simulink model "vehicle_hostmodel_2022b_v11"  (R2024b)
settings: Solver=ode4  StartTime=0.0  StopTime=inf  FixedStep=0.01  MaxStep=0.05  RelTol=1e-3
PreLoadFcn:
  | load("FInalGraph.mat")
model workspace (MAT data in the model file):
  G_final : digraph (value not decoded)
values from neighbouring files (symbols this model uses):
  ActorID = 0    [HelperSpeedActionAdapter.m]
  D = cross(B-A,C-A)    [HelperCalculateEgoRefPathInfo.m]
  L = zeros(N,1)    [HelperCalculateEgoRefPathInfo.m]
  psi_o = -1.185    [sensor.m]
  R = NaN(N,1)    [HelperCalculateEgoRefPathInfo.m]
  SceneInfo = [-32.1351766513 25.1612903226 -74.2242703533 -71.4592933948 -32.2887864823 26.2365591398 26.8509984639 27.0046082949 -32.7496159754 -72.380952381 -49.846390169 -49.3855606759 ... (30 elements, 10x3)]    [SceneLabels.mat]
  Ts = 0.05    [sensor.m]
undefined symbols (not defined in the file or in its folder): Acceleration, AngularVelocity, barrier_1, barrier_2, barrier_3, curvature, DefaultGear, DEND_B, DEND_S, DEND_T, direction, DiscIntNeverNeededParam, driving, finalint, goal1_coordinates, goal2_coordinates, goal3_coordinates, gradbp, latlongcoordinates, LF, LR, matlabshared, MAX_BRAKE, MAX_STEER, MAX_TORQUE, MCAR, MIN_BRAKE, MIN_STEER, MIN_TORQUE, NUMD_B, NUMD_S, NUMD_T, Pitch, Position, Roll, RRdamp, session, sigbuilder_block, STEER_RATIO, stopSign_ID, Tdead, thetaRefs, TL_ID, TrackWidth, ts, Vdead, Velocity, WB, xRef2s, Yaw, yRef2s
libraries: simulink x10, drivingscenarioandsensors x8, simulink_extras x4, drivingvehiclecontroller x2, trackingutilitieslib x2, robotalgslib x1, mpcadaslib x1, slpidlib x1, drivinglib x1, autolibshared x1, vehdynlibviscommon x1, vehdynlibsteering x1
(part 3 of 4)

== system vehicle_hostmodel_2022b_v11/Controllers/Subsystem2/Subsystem/Function-Call Subsystem ==
  CurrVelocity : Inport
  Relative Distance : Inport  Port=2
  function : TriggerPort  VariantControl=(inherit)  ShowOutputPort=on
  MATLAB Function1 : MATLAB Function  TreatAsAtomicUnit=on
  Saturation : Saturate  UpperLimit=0.3*9.8  LowerLimit=0
  BrakingAcc : Outport
  wires:
  CurrVelocity/1 -> MATLAB Function1/1(Vel)
  Relative Distance/1 -> MATLAB Function1/2(RelDist)
  MATLAB Function1/1(BrakingAcc) -> Saturation/1
  Saturation/1 -> BrakingAcc/1

== system vehicle_hostmodel_2022b_v11/Controllers/Subsystem2/Subsystem/Subsystem2 ==
  decc_cmd : Inport
  Constant1 : Constant  Value=MCAR
  Gain : Gain  Gain=1.1*MCAR
  Gain1 : Gain  Gain=1.2*0.3*2/2
  Gain2 : Gain  Gain=0.7*9.81
  Gain4 : Gain  Gain=-R/(7.05*0.8)
  Integrator : Integrator  ExternalReset=falling
  Square : Math  Operator=square
  Sum : Sum  Inputs=+++
  T_brake_cmd : Outport
  wires:
  Square/1 -> Gain1/1
  Integrator/1 -> Square/1  "v"
  Gain4/1 -> T_brake_cmd/1  "T_eng"
  Gain1/1 -> Sum/1  "F_aero"
  Gain2/1 -> Sum/2
  decc_cmd/1 -> Integrator/2, Integrator/1, Gain/1
  Sum/1 -> Gain4/1
  Gain/1 -> Sum/3
  Constant1/1 -> Gain2/1

== system vehicle_hostmodel_2022b_v11/Controllers/Subsystem2/Subsystem1/Subsystem2 ==
  acc_cmd : Inport
  decc_cmd : Inport  Port=2
  Subsystem : Subsystem
  Subsystem1 : Subsystem
  T_eng_cmd : Outport
  brake_cmd : Outport  Port=2
  wires:
  acc_cmd/1 -> Subsystem/1(acc_cmd)
  Subsystem/1(T_eng_cmd) -> T_eng_cmd/1
  decc_cmd/1 -> Subsystem1/1(decc_cmd)
  Subsystem1/1(T_brake_cmd) -> brake_cmd/1

== system vehicle_hostmodel_2022b_v11/Environment & Data/Sensors & Perception/Tracking/Subsystem1 ==
  In2 : Inport
  EgoV : Inport  Port=2
  Camera : drivingscenarioandsensors/Vision Detection Generator  SensorIndex=1  DetectorOutput=Objects only  UpdateInterval=0.1  LaneUpdateInterval=0.1  SensorLocation=[1.9 0]  Height=1.1  Yaw=0  Pitch=1  Roll=0  BusNameSource=Auto  BusName=BusObjectDetections  BusName2Source=Auto  BusName2=BusLaneDetections  MaxNumDetectionsSource=Property  MaxNumDetections=10  MaxNumLanesSource=Property  MaxNumLanes=30  DetectionCoordinates=Ego Cartesian  SimulateUsing=Interpreted execution  MaxRange=150  BoundingBoxAccuracy=5  ProcessNoiseIntensity=5  MaxSpeed=100  MaxAllowedOcclusion=0.5  MinObjectImageSize=[5 5]  DetectionProbability=0.9  FalsePositivesPerImage=0.1  MinLaneImageSize=[20 3]  LaneBoundaryAccuracy=3  HasNoise=on  InitialSeedSource=Repeatable  InitialSeed=0  UsedSeed=0  ActorProfilesSource=From Scenario Reader block  ActorProfilesParameters=driving.internal.ActorProfilesParameters  ActorProfilesExpression=[struct('ActorID',1,'ClassID',1,'Length',4.7,'Width',1.8,'Height',1.4,'OriginOffset',[-1.35 0 0],'MeshVertices',[3.7 0.9 0.857439446366782;3.7 -0.9 0.857439446366782;3.7 -0.9 0.314878892733564;3.7 0.9 0.314878892733564;3.7 0.9 0.857439446366782;2.525 0.9 0.993079584775086;2.525 -0.9 0.993079584775086;3.7 -0.9 0.857439446366782;1.82 0.72 1.4;0.41 0.72 1.4;0.41 -0.72 1.4;1.82 -0.72 1.4;-0.295 0.9 0.993079584775086;-1 0.9 0.857439446366782;-1 -0.9 0.857439446366782;-0.295 -0.9 0.993079584775086;3.7 0.9 0.857439446366782;3.7 0.9 0.314878892733564;2.525 0.9 0.314878892733564;2.525 0.9 0.993079584775086;2.525 0.9 0.993079584775086;2.525 0.9 0.314878892733564;-0.295 0.9 0.314878892733564;-0.295 0.9 0.993079584775086;-0.295 0.9 0.993079584775086;-0.295 0.9 0.314878892733564;-1 0.9 0.355570934256055;-1 0.9 0.857439446366782;2.525 0.9 0.993079584775086;-0.295 0.9 0.993079584775086;0.41 0.72 1.4;1.82 0.72 1.4;3.7 -0.9 0.857439446366782;3.7 -0.9 0.314878892733564;2.525 -0.9 0.314878892733564;2.525 -0.9 0.993079584775086;2.525 -0.9 0.993079584775086;2.525 -0.9 0.314878892733564;-0.295 -0.9 0.314878892733564;-0.295 -0.9 0.993079584775086;-0.295 -0.9 0.993079584775086;-0.295 -0.9 0.314878892733564;-1 -0.9 0.355570934256055;-1 -0.9 0.857439446366782;2.525 -0.9 0.993079584775086;-0.295 -0.9 0.993079584775086;0.41 -0.72 1.4;1.82 -0.72 1.4;-0.295 0.9 0.993079584775086;-0.295 -0.9 0.993079584775086;0.41 -0.72 1.4;0.41 0.72 1.4;2.525 -0.9 0.993079584775086;1.82 -0.72 1.4;1.82 0.72 1.4;2.525 0.9 0.993079584775086;-1 0.9 0.857439446366782;-1 0.9 0.355570934256055;-1 -0.9 0.355570934256055;-1 -0.9 0.857439446366782;3.7 0.9 0.314878892733564;3.7 -0.9 0.314878892733564;-0.295 -0.9 0.314878892733564;-0.295 0.9 0.314878892733564;-0.295 0.9 0.314878892733564;-1 0.9 0.355570934256055;-1 -0.9 0.355570934256055;-0.295 -0.9 0.314878892733564;0 -0.63 0;0 -0.87 0;0.191030206995054 -0.63 0.0601365173421445;0.191030206995054 -0.87 0.0601365173421445;0.309093367795925 -0.63 0.217575963708927;0.309093367795925 -0.87 0.217575963708927;0.309093367795925 -0.63 0.412181821758201;0.309093367795925 -0.87 0.412181821758201;0.191030206995054 -0.63 0.569621268124983;0.191030206995054 -0.87 0.569621268124983;0 -0.63 0.629757785467128;0 -0.87 0.629757785467128;-0.191030206995054 -0.63 0.569621268124983;-0.191030206995054 -0.87 0.569621268124983;-0.309093367795925 -0.63 0.412181821758201;-0.309093367795925 -0.87 0.412181821758201;-0.309093367795925 -0.63 0.217575963708927;-0.309093367795925 -0.87 0.217575963708927;-0.191030206995054 -0.63 0.0601365173421445;-0.191030206995054 -0.87 0.0601365173421445;0 -0.63 0;0 -0.87 0;0 -0.63 0;0.191030206995054 -0.63 0.0601365173421445;0.309093367795925 -0.63 0.217575963708927;0.309093367795925 -0.63 0.412181821758201;0.191030206995054 -0.63 0.569621268124983;0 -0.63 0.629757785467128;-0.191030206995054 -0.63 0.569621268124983;-0.309093367795925 -0.63 0.412181821758201;-0.309093367795925 -0.63 0.217575963708927;-0.191030206995054 -0.63 0.0601365173421445;0 -0.87 0;0.191030206995054 -0.87 0.0601365173421445;0.309093367795925 -0.87 0.217575963708927;0.309093367795925 -0.87 0.412181821758201;0.191030206995054 -0.87 0.569621268124983;0 -0.87 0.629757785467128;-0.191030206995054 -0.87 0.569621268124983;-0.309093367795925 -0.87 0.412181821758201;-0.309093367795925 -0.87 0.217575963708927;-0.191030206995054 -0.87 0.0601365173421445;0 0.87 0;0 0.63 0;0.191030206995054 0.87 0.0601365173421445;0.191030206995054 0.63 0.0601365173421445;0.309093367795925 0.87 0.217575963708927;0.309093367795925 0.63 0.217575963708927;0.309093367795925 0.87 0.412181821758201;0.309093367795925 0.63 0.412181821758201;0.191030206995054 0.87 0.569621268124983;0.191030206995054 0.63 0.569621268124983;0 0.87 0.629757785467128;0 0.63 0.629757785467128;-0.191030206995054 0.87 0.569621268124983;-0.191030206995054 0.63 0.569621268124983;-0.309093367795925 0.87 0.412181821758201;-0.309093367795925 0.63 0.412181821758201;-0.309093367795925 0.87 0.217575963708927;-0.309093367795925 0.63 0.217575963708927;-0.191030206995054 0.87 0.0601365173421445;-0.191030206995054 0.63 0.0601365173421445;0 ...(+3718 chars)],'MeshFaces',[1 2 3;3 4 1;5 6 7;7 8 5;9 10 11;11 12 9;13 14 15;15 16 13;17 18 19;19 20 17;21 22 23;23 24 21;25 26 27;27 28 25;29 30 31;31 32 29;33 34 35;35 36 33;37 38 39;39 40 37;41 42 43;43 44 41;45 46 47;47 48 45;49 50 51;51 52 49;53 54 55;55 56 53;57 58 59;59 60 57;61 62 63;63 64 61;65 66 67;67 68 65;69 71 72;72 70 69;71 73 74;74 72 71;73 75 76;76 74 73;75 77 78;78 76 75;77 79 80;80 78 77;79 81 82;82 80 79;81 83 84;84 82 81;83 85 86;86 84 83;85 87 88;88 86 85;87 89 90;90 88 87;91 92 93;91 93 94;91 94 95;91 95 96;91 96 97;91 97 98;91 98 99;91 99 100;101 102 103;101 103 104;101 104 105;101 105 106;101 106 107;101 107 108;101 108 109;101 109 110;111 113 114;114 112 111;113 115 116;116 114 113;115 117 118;118 116 115;117 119 120;120 118 117;119 121 122;122 120 119;121 123 124;124 122 121;123 125 126;126 124 123;125 127 128;128 126 125;127 129 130;130 128 127;129 131 132;132 130 129;133 134 135;133 135 136;133 136 137;133 137 138;133 138 139;133 139 140;133 140 141;133 141 142;143 144 145;143 145 146;143 146 147;143 147 148;143 148 149;143 149 150;143 150 151;143 151 152;153 155 156;156 154 153;155 157 158;158 156 155;157 159 160;160 158 157;159 161 162;162 160 159;161 163 164;164 162 161;163 165 166;166 164 163;165 167 168;168 166 165;167 169 170;170 168 167;169 171 172;172 170 169;171 173 174;174 172 171;175 176 177;175 177 178;175 178 179;175 179 180;175 180 181;175 181 182;175 182 183;175 183 184;185 186 187;185 187 188;185 188 189;185 189 190;185 190 191;185 191 192;185 192 193;185 193 194;195 197 198;198 196 195;197 199 200;200 198 197;199 201 202;202 200 199;201 203 204;204 202 201;203 205 206;206 204 203;205 207 208;208 206 205;207 209 210;210 208 207;209 211 212;212 210 209;211 213 214;214 212 211;213 215 216;216 214 213;217 218 219;217 219 220;217 220 221;217 221 222;217 222 223;217 223 224;217 224 225;217 225 226;227 228 229;227 229 230;227 230 231;227 231 232;227 232 233;227 233 234;227 234 235;227 235 236],'RCSPattern',[10 10;10 10],'RCSAzimuthAngles',[-180 180],'RCSElevationAngles',[-90 90]); struct('ActorID',2,'ClassID',7,'Length',0.7,'Width',0.2,'Height',0.1,'OriginOffset',[0 0 0],'MeshVertices',[0.35 -0.1 0.1;0.35 0.1 0.1;-0.35 0.1 0.1;-0.35 -0.1 0.1;0.35 -0.1 0;0.35 0.1 0;-0.35 0.1 0;-0.35 -0.1 0],'MeshFaces',[6 2 1;1 5 6;8 4 3;3 7 8;6 7 3;3 2 6;5 1 4;4 8 5;4 1 2;2 3 4;7 6 5;5 8 7],'RCSPattern',[10 10;10 10],'RCSAzimuthAngles',[-180 180],'RCSElevationAngles',[-90 90])]  Intrinsics=driving.internal.cameraIntrinsics('FocalLength',[800 800],'PrincipalPoint',[320 240],'ImageSize',[480 640],'RadialDistortion',[0 0],'TangentialDistortion',[0 0],'Skew',0)
  Detection Concatenation : trackingutilitieslib/Detection Concatenation  NumInputs=3  BusNameSource=Auto  BusName=BusDetectionConcatenation  SimulateUsing=Interpreted execution
  Lidar Point Cloud Generator : drivingscenarioandsensors/Lidar Point Cloud Generator  SensorIndex=2  UpdateInterval=0.1  SensorLocation=[1.5 0]  Height=1.6  Yaw=0  Pitch=0  Roll=0  DetectionCoordinates=Ego Cartesian  HasEgoVehicle=on  EgoVehicleActorID=1  HasRoadsInputPort=on  ActorProfilesSource=From Scenario Reader block  ActorProfilesVariableName=actor_profiles  MaxRange=120  RangeAccuracy=0.002  AzimuthResolution=0.16  ElevationResolution=1.25  AzimuthLimits=[-60 60]  ElevationLimits=[ -20, 20 ]  HasNoise=on
  Lidar Point Cloud Generator1 : drivingscenarioandsensors/Lidar Point Cloud Generator  SensorIndex=3  UpdateInterval=0.1  SensorLocation=[1.5 0]  Height=1.6  Yaw=0  Pitch=0  Roll=0  DetectionCoordinates=Ego Cartesian  HasEgoVehicle=on  EgoVehicleActorID=1  HasRoadsInputPort=on  ActorProfilesSource=From Scenario Reader block  ActorProfilesVariableName=actor_profiles  MaxRange=120  RangeAccuracy=0.002  AzimuthResolution=0.16  ElevationResolution=1.25  AzimuthLimits=[60 180]  ElevationLimits=[ -20, 20 ]  HasNoise=on
  Lidar Point Cloud Generator2 : drivingscenarioandsensors/Lidar Point Cloud Generator  SensorIndex=4  UpdateInterval=0.1  SensorLocation=[1.5 0]  Height=1.6  Yaw=0  Pitch=0  Roll=0  DetectionCoordinates=Ego Cartesian  HasEgoVehicle=on  EgoVehicleActorID=1  HasRoadsInputPort=on  ActorProfilesSource=From Scenario Reader block  ActorProfilesVariableName=actor_profiles  MaxRange=120  RangeAccuracy=0.002  AzimuthResolution=0.16  ElevationResolution=1.25  AzimuthLimits=[-180 -60]  ElevationLimits=[ -20, 20 ]  HasNoise=on
  Camera Detections : Outport
  Radar detections : Outport  Port=2
  wires:
  EgoV/1 -> Lidar Point Cloud Generator1/2, Lidar Point Cloud Generator/2, Lidar Point Cloud Generator2/2
  Lidar Point Cloud Generator1/1 -> Detection Concatenation/2  "Lidar Detections"
  Lidar Point Cloud Generator2/1 -> Detection Concatenation/3  "Lidar Detections"
  Detection Concatenation/1 -> Radar detections/1
  Camera/1 -> Camera Detections/1  "Camera Detections"
  In2/1 -> Camera/1, Lidar Point Cloud Generator/1, Lidar Point Cloud Generator1/1, Lidar Point Cloud Generator2/1
  Lidar Point Cloud Generator/1 -> Detection Concatenation/1  "Lidar Detections"

== system vehicle_hostmodel_2022b_v11/Environment & Data/Visualisation & Data/Positions and States /Traffic Light Sensor ==
  note: Traffic Light Sensor
  TL_id : Inport
  Bus Creator : BusCreator  Inputs=2
  LightConfiguration : Constant  Value=TrafficLightSensorModeSelection
  Traffic Light Switching Logic : Stateflow chart  TreatAsAtomicUnit=on
  TL_State : Outport
  wires:
  LightConfiguration/1 -> Traffic Light Switching Logic/1(LightConfig)
  TL_id/1 -> Traffic Light Switching Logic/2(TL_id)
  Bus Creator/1 -> TL_State/1
  Traffic Light Switching Logic/2(trafficLight) -> Bus Creator/1
  Traffic Light Switching Logic/1(TL_ID) -> Bus Creator/2

== system vehicle_hostmodel_2022b_v11/Reference Data1/Subsystem1/Subsystem2/Subsystem ==
  note: Select method to calculate theta
  Integrator : Inport
  Curvature : Lookup_n-D  NumberOfTableDimensions=1  BreakpointsForDimension1=gradbp  Table=curvature  InternalRulePriority=Speed  RndMeth=Simplest
  Direction : Lookup_n-D  NumberOfTableDimensions=1  BreakpointsForDimension1=gradbp  Table=direction  InternalRulePriority=Speed  RndMeth=Simplest
  From Workspace1 : FromWorkspace  VariableName=yRef2  SampleTime=-1
  From Workspace2 : FromWorkspace  VariableName=xRef2  SampleTime=-1
  From Workspace3 : FromWorkspace  VariableName=gradbp  SampleTime=-1
  Goto : Goto  Commented=on  GotoTag=xRef  TagVisibility=global
  Goto1 : Goto  Commented=on  GotoTag=yRef  TagVisibility=global
  Matrix Concatenate : Concatenate  Mode=Multidimensional array  ConcatenateDimension=2
  Mux : Mux  Inputs=3
  Switch Case : SwitchCase
  Theta : Subsystem  Variant=on  VariantControlMode=label  LabelModeActiveChoice=thetaLookUpTable
  X Ref : Lookup_n-D  NumberOfTableDimensions=1  BreakpointsForDimension1=gradbp  Table=xRef2s  InternalRulePriority=Speed  RndMeth=Simplest
  Y Ref : Lookup_n-D  NumberOfTableDimensions=1  BreakpointsForDimension1Source=Input port  BreakpointsForDimension1=gradbp  TableSource=Input port  Table=yRef2s  InternalRulePriority=Speed  RndMeth=Simplest
      settings: InputPortMap=u0,p221,p5
  Out1 : Outport
  Out2 : Outport  Port=2
  CurvatureO : Outport  Port=3
  DirectionO : Outport  Port=4
  finalint : Outport  Port=5
  wires:
  Direction/1 -> DirectionO/1
  Y Ref/1 -> Theta/1(y), Mux/2, Goto1/1
  Theta/1(theta) -> Mux/3
  X Ref/1 -> Theta/2(x), Mux/1, Goto/1
  Matrix Concatenate/1 -> Out1/1
  Curvature/1 -> CurvatureO/1
  Mux/1 -> Out2/1
  From Workspace1/1 -> Y Ref/2, Matrix Concatenate/2
  From Workspace2/1 -> Matrix Concatenate/1
  From Workspace3/1 -> Y Ref/3
  Integrator/1 -> Direction/1, Curvature/1, Theta/3(dis), Y Ref/1, X Ref/1

== system vehicle_hostmodel_2022b_v11/Reference Data1/Subsystem1/Subsystem3/Subsystem ==
  note: Select method to calculate theta
  xd : Inport
  yd : Inport  Port=2
  Integrator : Inport  Port=3
  Add Constant : Bias  Bias=6.5  SaturateOnIntegerOverflow=off
  Curvature : Lookup_n-D  NumberOfTableDimensions=1  BreakpointsForDimension1=gradbp  Table=curvature  InternalRulePriority=Speed  RndMeth=Simplest
  Direction : Lookup_n-D  NumberOfTableDimensions=1  BreakpointsForDimension1=gradbp  Table=direction  InternalRulePriority=Speed  RndMeth=Simplest
  From Workspace1 : FromWorkspace  VariableName=yRef2  SampleTime=-1
  From Workspace2 : FromWorkspace  VariableName=xRef2  SampleTime=-1
  From Workspace3 : FromWorkspace  VariableName=gradbp  SampleTime=-1
  Goto : Goto  Commented=on  GotoTag=xRef  TagVisibility=global
  Goto1 : Goto  Commented=on  GotoTag=yRef  TagVisibility=global
  Matrix Concatenate : Concatenate  Mode=Multidimensional array  ConcatenateDimension=2
  Mux : Mux  Inputs=3
  Theta : Subsystem  Variant=on  VariantControlMode=label  LabelModeActiveChoice=thetaLookUpTable
  X Ref : Lookup_n-D  NumberOfTableDimensions=1  BreakpointsForDimension1Source=Input port  BreakpointsForDimension1=gradbp  TableSource=Input port  Table=xRef2s  InternalRulePriority=Speed  RndMeth=Simplest
      settings: InputPortMap=u0,p221,p5
  Y Ref : Lookup_n-D  NumberOfTableDimensions=1  BreakpointsForDimension1Source=Input port  BreakpointsForDimension1=gradbp  TableSource=Input port  Table=yRef2s  InternalRulePriority=Speed  RndMeth=Simplest
      settings: InputPortMap=u0,p221,p5
  Out1 : Outport
  Out2 : Outport  Port=2
  CurvatureO : Outport  Port=3
  DirectionO : Outport  Port=4
  wires:
  Direction/1 -> DirectionO/1
  Theta/1(theta) -> Mux/3
  Matrix Concatenate/1 -> Out1/1
  Curvature/1 -> CurvatureO/1
  Mux/1 -> Out2/1
  From Workspace1/1 -> Add Constant/1, Matrix Concatenate/2
  From Workspace2/1 -> X Ref/2, Matrix Concatenate/1
  From Workspace3/1 -> Y Ref/3, X Ref/3
  X Ref/1 -> Theta/2(x), Mux/1
  Add Constant/1 -> Y Ref/2
  Y Ref/1 -> Theta/1(y), Mux/2
  Integrator/1 -> Direction/1, Curvature/1, Theta/3(dis), Y Ref/1, X Ref/1

== system vehicle_hostmodel_2022b_v11/Reference Data1/Subsystem2/Subsystem/Theta ==
  note: 1) Add Subsystem or Model blocks as valid variant choices.
      | 2) You cannot connect blocks at this level. At simulation, connectivity is automatically
      | determined, based on the active variant and port name matching.
  y : Inport
  x : Inport  Port=2
  dis : Inport  Port=3
  thetaBlocks : Subsystem  VariantControl=thetaSimulinkBlock
  thetaLt : Subsystem  VariantControl=thetaLookUpTable
  theta : Outport

== system vehicle_hostmodel_2022b_v11/Reference Data1/Subsystem3/Subsystem/Theta ==
  note: 1) Add Subsystem or Model blocks as valid variant choices.
      | 2) You cannot connect blocks at this level. At simulation, connectivity is automatically
      | determined, based on the active variant and port name matching.
  y : Inport
  x : Inport  Port=2
  dis : Inport  Port=3
  thetaBlocks : Subsystem  VariantControl=thetaSimulinkBlock
  thetaLt : Subsystem  VariantControl=thetaLookUpTable
  theta : Outport

== system vehicle_hostmodel_2022b_v11/Controllers/Subsystem2/Subsystem1/Subsystem2/Subsystem ==
  acc_cmd : Inport
  Constant1 : Constant  Value=MCAR
  Gain : Gain  Gain=1.1*MCAR
  Gain1 : Gain  Gain=1.2*0.3*2/2
  Gain2 : Gain  Gain=0.7*9.81
  Gain4 : Gain  Gain=R/(7.05*0.8)
  Integrator : Integrator  ExternalReset=falling
  Square : Math  Operator=square
  Sum : Sum  Inputs=+++
  T_eng_cmd : Outport
  wires:
  Constant1/1 -> Gain2/1
  Gain/1 -> Sum/3
  Sum/1 -> Gain4/1
  acc_cmd/1 -> Gain/1, Integrator/2, Integrator/1
  Gain2/1 -> Sum/2
  Gain1/1 -> Sum/1  "F_aero"
  Gain4/1 -> T_eng_cmd/1  "T_eng"
  Integrator/1 -> Square/1  "v"
  Square/1 -> Gain1/1

== system vehicle_hostmodel_2022b_v11/Controllers/Subsystem2/Subsystem1/Subsystem2/Subsystem1 ==
  decc_cmd : Inport
  Constant1 : Constant  Value=MCAR
  Gain : Gain  Gain=1.1*MCAR
  Gain1 : Gain  Gain=1.2*0.3*2/2
  Gain2 : Gain  Gain=0.7*9.81
  Gain4 : Gain  Gain=-R/(7.05*0.8)
  Integrator : Integrator  ExternalReset=falling
  Square : Math  Operator=square
  Sum : Sum  Inputs=+++
  T_brake_cmd : Outport
  wires:
  Square/1 -> Gain1/1
  Integrator/1 -> Square/1  "v"
  Gain4/1 -> T_brake_cmd/1  "T_eng"
  Gain1/1 -> Sum/1  "F_aero"
  Gain2/1 -> Sum/2
  decc_cmd/1 -> Integrator/2, Integrator/1, Gain/1
  Sum/1 -> Gain4/1
  Gain/1 -> Sum/3
  Constant1/1 -> Gain2/1

== system vehicle_hostmodel_2022b_v11/Reference Data1/Subsystem1/Subsystem2/Subsystem/Theta ==
  note: 1) Add Subsystem or Model blocks as valid variant choices.
      | 2) You cannot connect blocks at this level. At simulation, connectivity is automatically
      | determined, based on the active variant and port name matching.
  y : Inport
  x : Inport  Port=2
  dis : Inport  Port=3
  thetaBlocks : Subsystem  VariantControl=thetaSimulinkBlock
  thetaLt : Subsystem  VariantControl=thetaLookUpTable
  theta : Outport

== system vehicle_hostmodel_2022b_v11/Reference Data1/Subsystem1/Subsystem3/Subsystem/Theta ==
  note: 1) Add Subsystem or Model blocks as valid variant choices.
      | 2) You cannot connect blocks at this level. At simulation, connectivity is automatically
      | determined, based on the active variant and port name matching.
  y : Inport
  x : Inport  Port=2
  dis : Inport  Port=3
  thetaBlocks : Subsystem  VariantControl=thetaSimulinkBlock
  thetaLt : Subsystem  VariantControl=thetaLookUpTable
  theta : Outport

== system vehicle_hostmodel_2022b_v11/Reference Data1/Subsystem2/Subsystem/Theta/thetaBlocks ==
  note: theta calculated from Simulink blocks
  y : Inport
  x : Inport  Port=2
  dis : Inport  Port=3
  Atan2 : Trigonometry  Operator=atan2  ApproximationMethod=CORDIC
  Difference : simulink/Discrete/Difference  ICPrevInput=0.0  OutMin=[]  OutMax=[]  OutDataType=fixdt(1, 16)  OutScaling=2^-10  DoSatur=off
  Difference1 : simulink/Discrete/Difference  ICPrevInput=0.0  OutMin=[]  OutMax=[]  OutDataType=fixdt(1, 16)  OutScaling=2^-10  DoSatur=off
  IC : InitialCondition  Value=psi_o
  Radians to Degrees : simulink_extras/Transformations/Radians to Degrees
  Terminator : Terminator
  theta : Outport
  wires:
  IC/1 -> Radians to Degrees/1
  Atan2/1 -> IC/1
  dis/1 -> Terminator/1
  x/1 -> Difference1/1
  y/1 -> Difference/1
  Radians to Degrees/1 -> theta/1
  Difference/1 -> Atan2/1
  Difference1/1 -> Atan2/2

== system vehicle_hostmodel_2022b_v11/Reference Data1/Subsystem2/Subsystem/Theta/thetaLt ==
  note: Check out the script "setUpModel" to understand how we have calculated theta
  note: theta based on lookup table
  y : Inport
  x : Inport  Port=2
  dis : Inport  Port=3
  Terminator : Terminator
  Terminator1 : Terminator
  Theta Ref : Lookup_n-D  NumberOfTableDimensions=1  BreakpointsForDimension1=gradbp  Table=thetaRefs  InternalRulePriority=Speed  RndMeth=Simplest
  theta : Outport
  wires:
  Theta Ref/1 -> theta/1
  dis/1 -> Theta Ref/1
  x/1 -> Terminator1/1
  y/1 -> Terminator/1

== system vehicle_hostmodel_2022b_v11/Reference Data1/Subsystem3/Subsystem/Theta/thetaBlocks ==
  note: theta calculated from Simulink blocks
  y : Inport
  x : Inport  Port=2
  dis : Inport  Port=3
  Atan2 : Trigonometry  Operator=atan2  ApproximationMethod=CORDIC
  Difference : simulink/Discrete/Difference  ICPrevInput=0.0  OutMin=[]  OutMax=[]  OutDataType=fixdt(1, 16)  OutScaling=2^-10  DoSatur=off
  Difference1 : simulink/Discrete/Difference  ICPrevInput=0.0  OutMin=[]  OutMax=[]  OutDataType=fixdt(1, 16)  OutScaling=2^-10  DoSatur=off
  IC : InitialCondition  Value=psi_o
  Radians to Degrees : simulink_extras/Transformations/Radians to Degrees
  Terminator : Terminator
  theta : Outport
  wires:
  IC/1 -> Radians to Degrees/1
  Atan2/1 -> IC/1
  dis/1 -> Terminator/1
  x/1 -> Difference1/1
  y/1 -> Difference/1
  Radians to Degrees/1 -> theta/1
  Difference/1 -> Atan2/1
  Difference1/1 -> Atan2/2

== system vehicle_hostmodel_2022b_v11/Reference Data1/Subsystem3/Subsystem/Theta/thetaLt ==
  note: Check out the script "setUpModel" to understand how we have calculated theta
  note: theta based on lookup table
  y : Inport
  x : Inport  Port=2
  dis : Inport  Port=3
  Terminator : Terminator
  Terminator1 : Terminator
  Theta Ref : Lookup_n-D  NumberOfTableDimensions=1  BreakpointsForDimension1=gradbp  Table=thetaRefs  InternalRulePriority=Speed  RndMeth=Simplest
  theta : Outport
  wires:
  Theta Ref/1 -> theta/1
  dis/1 -> Theta Ref/1
  x/1 -> Terminator1/1
  y/1 -> Terminator/1

== system vehicle_hostmodel_2022b_v11/Reference Data1/Subsystem1/Subsystem2/Subsystem/Theta/thetaBlocks ==
  note: theta calculated from Simulink blocks
  y : Inport
  x : Inport  Port=2
  dis : Inport  Port=3
  Atan2 : Trigonometry  Operator=atan2  ApproximationMethod=CORDIC
  Difference : simulink/Discrete/Difference  ICPrevInput=0.0  OutMin=[]  OutMax=[]  OutDataType=fixdt(1, 16)  OutScaling=2^-10  DoSatur=off
  Difference1 : simulink/Discrete/Difference  ICPrevInput=0.0  OutMin=[]  OutMax=[]  OutDataType=fixdt(1, 16)  OutScaling=2^-10  DoSatur=off
  IC : InitialCondition  Value=psi_o
  Radians to Degrees : simulink_extras/Transformations/Radians to Degrees
  Terminator : Terminator
  theta : Outport
  wires:
  IC/1 -> Radians to Degrees/1
  Atan2/1 -> IC/1
  dis/1 -> Terminator/1
  x/1 -> Difference1/1
  y/1 -> Difference/1
  Radians to Degrees/1 -> theta/1
  Difference/1 -> Atan2/1
  Difference1/1 -> Atan2/2

== system vehicle_hostmodel_2022b_v11/Reference Data1/Subsystem1/Subsystem2/Subsystem/Theta/thetaLt ==
  note: Check out the script "setUpModel" to understand how we have calculated theta
  note: theta based on lookup table
  y : Inport
  x : Inport  Port=2
  dis : Inport  Port=3
  Terminator : Terminator
  Terminator1 : Terminator
  Theta Ref : Lookup_n-D  NumberOfTableDimensions=1  BreakpointsForDimension1=gradbp  Table=thetaRefs  InternalRulePriority=Speed  RndMeth=Simplest
  theta : Outport
  wires:
  Theta Ref/1 -> theta/1
  dis/1 -> Theta Ref/1
  x/1 -> Terminator1/1
  y/1 -> Terminator/1

== system vehicle_hostmodel_2022b_v11/Reference Data1/Subsystem1/Subsystem3/Subsystem/Theta/thetaBlocks ==
  note: theta calculated from Simulink blocks
  y : Inport
  x : Inport  Port=2
  dis : Inport  Port=3
  Atan2 : Trigonometry  Operator=atan2  ApproximationMethod=CORDIC
  Difference : simulink/Discrete/Difference  ICPrevInput=0.0  OutMin=[]  OutMax=[]  OutDataType=fixdt(1, 16)  OutScaling=2^-10  DoSatur=off
  Difference1 : simulink/Discrete/Difference  ICPrevInput=0.0  OutMin=[]  OutMax=[]  OutDataType=fixdt(1, 16)  OutScaling=2^-10  DoSatur=off
  IC : InitialCondition  Value=psi_o
  Radians to Degrees : simulink_extras/Transformations/Radians to Degrees
  Terminator : Terminator
  theta : Outport
  wires:
  IC/1 -> Radians to Degrees/1
  Atan2/1 -> IC/1
  dis/1 -> Terminator/1
  x/1 -> Difference1/1
  y/1 -> Difference/1
  Radians to Degrees/1 -> theta/1
  Difference/1 -> Atan2/1
  Difference1/1 -> Atan2/2

== system vehicle_hostmodel_2022b_v11/Reference Data1/Subsystem1/Subsystem3/Subsystem/Theta/thetaLt ==
  note: Check out the script "setUpModel" to understand how we have calculated theta
  note: theta based on lookup table
  y : Inport
  x : Inport  Port=2
  dis : Inport  Port=3
  Terminator : Terminator
  Terminator1 : Terminator
  Theta Ref : Lookup_n-D  NumberOfTableDimensions=1  BreakpointsForDimension1=gradbp  Table=thetaRefs  InternalRulePriority=Speed  RndMeth=Simplest
  theta : Outport
  wires:
  Theta Ref/1 -> theta/1
  dis/1 -> Theta Ref/1
  x/1 -> Terminator1/1
  y/1 -> Terminator/1

== matlab function vehicle_hostmodel_2022b_v11/Environment & Data/Visualisation & Data/Positions and States /MATLAB Function2 ==
  data: Actors input; ss_poses output; ss_State input

function ss_poses = findssposes(Actors, ss_State)

n=length(ss_State);
ss_poses=zeros(n,4);
indices=zeros(n,1);
ID=zeros(length(Actors),1);

for i=1:length(Actors)
 ID(i)=Actors(i).ActorID;
end

indices=find(ismember(ID,ss_State));
if(~isempty(indices))
    
    for i=1:n
        ss_poses(i,:)=([Actors(indices(i)).Position(:)',ss_State(i)]);
    end
end

ss_poses(ss_poses==0)=NaN;






% ss1_poses=zeros(1,4);
% ss2_poses=zeros(1,4);
% for i=1:length(Actors)
%     ID=Actors(i).ActorID;
%     
%     if(ID==ss1_State(1))
%         ss1_poses=[Actors(i).Position(:)',ss1_State(1)];
%     elseif ID== (ss1_State(2))
%         ss2_poses=[Actors(i).Position(:)',ss1_State(2)];
%     
%     end
%   
% end
% ss1_poses(ss1_poses==0)=NaN;   
% ss2_poses(ss2_poses==0)=NaN;

== matlab function vehicle_hostmodel_2022b_v11/Environment & Data/Visualisation & Data/Positions and States /MATLAB Function1 ==
  data: Actors input; TL_poses output; TL_State input

function TL_poses = findTLposes(Actors, TL_State)
n=length(TL_State);
TL_poses=zeros(n/2,5);
indices=zeros(n/2,1);
ID=zeros(length(Actors),1);

for i=1:length(Actors)
 ID(i)=Actors(i).ActorID;
end

indices=find(ismember(ID,TL_State(n/2+1:end)));
if (~isempty(indices))

    for i=1:n/2
        TL_poses(i,:)=([Actors(indices(i)).Position(:)',TL_State(i),ID(indices(i))]);

    end
end
TL_poses(TL_poses==0)=NaN;

== stateflow chart vehicle_hostmodel_2022b_v11/Environment & Data/Visualisation & Data/Positions and States /Traffic Light Sensor/Traffic Light Switching Logic ==
  state STEADYRED
    entry:
    trafficLight(:)= Red; TL_ID=TL_id;
  state STEADYGREEN
    entry:
    trafficLight(:)= Green; TL_ID=TL_id;
  state START
    entry:
    trafficLight=TL_id;
    trafficLight(:)= Black;TL_ID=TL_id;
  state TRAFFICLIGHT_ODDYELLOW_EVENRED
    entry:
    trafficLight(1:2:end)=Yellow;TL_ID(1:2:end)=TL_id(1:2:end);
    trafficLight(2:2:end) = Red;TL_ID(2:2:end)=TL_id(2:2:end);
  state TRAFFICLIGHT_ODDGREEN_EVENRED
    entry:
    trafficLight(1:2:end)=Green;TL_ID(1:2:end)=TL_id(1:2:end);
    trafficLight(2:2:end) = Red;TL_ID(2:2:end)=TL_id(2:2:end);
  state TRAFFICLIGHT_ODDRED_EVENYELLOW
    entry:
    trafficLight(1:2:end)=Red;TL_ID(1:2:end)=TL_id(1:2:end);
    trafficLight(2:2:end) = Yellow;TL_ID(2:2:end)=TL_id(2:2:end);
  state TRAFFICLIGHT_ODDRED_EVENGREEN
    entry:
    trafficLight(1:2:end)=Red;TL_ID(1:2:end)=TL_id(1:2:end);
    trafficLight(2:2:end) = Green;TL_ID(2:2:end)=TL_id(2:2:end);
  (default) -> START
  START -> STEADYGREEN [order 3] : [LightConfig==1]
  START -> STEADYRED [order 1] : [LightConfig==2]
  START -> TRAFFICLIGHT_ODDGREEN_EVENRED [order 2] : [LightConfig ==3]
  TRAFFICLIGHT_ODDGREEN_EVENRED -> TRAFFICLIGHT_ODDYELLOW_EVENRED : after(4,sec)
  TRAFFICLIGHT_ODDYELLOW_EVENRED -> TRAFFICLIGHT_ODDRED_EVENGREEN : after(1,sec)
  TRAFFICLIGHT_ODDRED_EVENYELLOW -> TRAFFICLIGHT_ODDGREEN_EVENRED : after(1,sec)
  TRAFFICLIGHT_ODDRED_EVENGREEN -> TRAFFICLIGHT_ODDRED_EVENYELLOW : after(4,sec)
  data: Green constant double =3; Red constant double =1; Yellow constant double =2; LightConfig input; TL_id input; Black constant double =0; TL_ID output; trafficLight output

== matlab function vehicle_hostmodel_2022b_v11/Environment & Data/Sensors & Perception/MATLAB Function ==
  data: SceneID output; ObjRelVel output; SceneRelVel output; SceneDist output; ObjectDist output; ObjAhead output; SDist input; Tracking input; SceneAhead output; RelVelmin output; RelDistmin output; Trans input; ObjectMIO_Position output
function [SceneID,ObjRelVel,SceneRelVel,SceneDist,ObjectDist,ObjAhead,SceneAhead,RelVelmin,RelDistmin,ObjectMIO_Position]= SFDetections(SDist,Tracking, Trans)
ObjectID = zeros(20,1);
TrackPos = zeros(3,20);
TrackVel = zeros(3,20);
ObjectDist = 100; % zeros(20,1);
SceneDist = 100;
ObjRelVel = 10;
SceneRelVel = 10;
% ScenePos = [0 0];
ObjAhead = 0;
SceneAhead = 0;
SceneID = 0;
TracksNum = Tracking.NumTracks;
ObjectMIO_Position = zeros(3,1);


for t = 1:TracksNum
    ObjectID(t) = Tracking.Tracks(t).ObjectClassID;
    TrackPos(:,t) = Tracking.Tracks(t).State(1:2:5);
    TrackVel(:,t) = Tracking.Tracks(t).State(2:2:6);
   
    if TrackPos(2,t) < 1 && TrackPos(2,t) > -4 && abs(TrackPos(1,t)) <= SDist
        
        if ObjectID(t) >= 7 % 7=SS 8=TL 9=RA 10=RRC % labels {1,2,3,4} => {'TrafficLight','StopSign','RailRoadCrossing','RoundAbout'};
            SceneAhead = 1;
            SceneDist = min(SceneDist,TrackPos(1,t));
            if TrackPos(1,t) <= SceneDist
                % ScenePos = TrackPos(1:2,t)';
                SceneRelVel = TrackVel(1,t);
                SceneID = ObjectID(t);
            end
        end

        if ObjectID(t) < 7 && ObjectID(t) > 0
            ObjAhead = 1;
            ObjectDist = min(ObjectDist,TrackPos(1,t));
            ObjectMIO_Position(:,1) = TrackPos(:,t);

            if TrackPos(1,t) <= ObjectDist
                ObjRelVel = TrackVel(1,t);
                ObjID = ObjectID(t);
            end
        end

    end
    
end

if Trans == 1  % ObjectDist <= SceneDist
    RelVelmin = ObjRelVel;
    RelDistmin = ObjectDist;
else
    RelVelmin = min(SceneRelVel,ObjRelVel);
    RelDistmin = min(SceneDist,ObjectDist);
end

== matlab function vehicle_hostmodel_2022b_v11/Vehicle Dynamics/Info2ActorState/MATLAB Function ==
  data: X input; Position output; Y input; Z input
function Position = fcn(X, Y, Z)

Position = [X Y, Z];

== matlab function vehicle_hostmodel_2022b_v11/Subsystem/PathPlanner/MATLAB Function4 ==
  data: Distance output; output input; CurrentPose input; point output
function [Distance,point] = d2f(output,CurrentPose)



%Distance = norm(output(end,:) - CurrentPose(1:2)');
Distance= output(end,1)- CurrentPose(1);
point=output(end,:);

end

%Distance = sqrt(CurrentPose(1)-output(99,1))^2 + (CurrentPose(2)-output(99,2)^2);
%CurrentPose
%output=zeros(99,2);
%lastPoint = output(end,:);
%dx = lastPoint(1) - x;
%dx= output(end,1)-x;
%dy = output(end,2) - y;
%distance = sqrt(dx^2 + dy^2);

== matlab function vehicle_hostmodel_2022b_v11/Environment & Data/Sensors & Perception/MATLAB Function1 ==
  data: EVpos input; yaw input; SceneID input; SceneInfo input; SDir output; SDist input; D2S output
function [SDir,D2S] = SceneFinder(EVpos,yaw, SceneID, SceneInfo, SDist)
D2S = zeros(10,1);
    % dist = zeros(1,length(SceneLocations));
    for j = 1:length(SceneInfo(:,1))
        distXY = SceneInfo(j,1:2) - EVpos(1:2);
        D2S(j) = norm(distXY);
        
%         if (D2S <= SDist)
%             Scene = SceneInfo(j,3); % labels {1,2,3,4} => {'TrafficLight','StopSign','RailRoadCrossing','RoundAbout'};
%             angl = atan2d(distXY(2),distXY(1));
%             angl = angl - yaw;
% %             rot = [cosd(angl) -sind(angl);sind(angl) cosd(angl)];
% %             distXY = rot*distXY';
% %             angl = atan2d(distXY(2),distXY(1));
%             
%             if angl < 0
%                 angl = angl + 360;
%             end
% 
%             if (angl > 315) || (angl <= 45) 
%                 SDir = "N";
%             elseif (angl > 225) && (angl <= 315)
%                 SDir = "E";
%             elseif (angl > 135) && (angl <= 225)
%                 SDir = "S";
%                 D2S = 1000;
%                 angl = 1000;
%                 Scene = 0;
%             elseif (angl > 45) && (angl <= 135)
%                 SDir = "W";
%             else
%                 SDir = "Error";
%             end
%             break
%         else
%             Scene = 0;
%             SDir = " ";
%             angl = 1000;
%             D2S = 1000;
%         end

    end
[val,indx] = min(D2S);

== matlab function vehicle_hostmodel_2022b_v11/Subsystem/Function-Call Subsystem/MATLAB Function2 ==
  data: EgoPosition input; MIOPos input; curvature input; MIOVel input; V_i input; xd output; yd output; laneL input; laneR input; V_desired input; LCinProgress output
function [xd,yd,LCinProgress] = traj(EgoPosition,MIOPos,curvature,MIOVel, V_i, laneL, laneR, V_desired)
Vx_i =0;Vx_f=0;Vy_i=0;Vy_f=0;Ax_i=0;Ax_f=0;Ay_i=0;Ay_f=0;T_i=0;T_f=0;V_f=0;A_f=0;x_set=0;y_set=0;theta4=0;

P = zeros(6,6);
% xq = zeros(1,size(RefPath,1)); yq = zeros(1,size(RefPath,2));
EgoPosition(1,2)=-EgoPosition(1,2)
x_init= EgoPosition(1,1)+0.5; y_init = EgoPosition(1,2)-0.8;
% xq = RefPath(:,1)'; 
% yq = RefPath(:,2)';
num_foc_t = 98;
V_max= V_desired; ad_n=0; vd_n=MIOVel; wd_n=vd_n*curvature;
lane_width = 3.6 * (laneL-laneR); % +1 if left of current lane and -1 if right of current lane
xd = zeros(num_foc_t+1,1); 
yd = zeros(num_foc_t+1,1);
xf =0; 
yf = 0;

    %xf = [EgoPosition(1,1)+ MIOPos(1) ]; yf = [ EgoPosition(1,2)+ MIOPos(2) + lane_width];  
    xf = [EgoPosition(1,1)+ 40 ]; yf = [ EgoPosition(1,2)+ 1.1*lane_width]; % 80
    V_f = V_max;
    W_f = V_f*curvature;
    A_f = 0;

    %dist2crash = sqrt((x_init-MIOPos(1))^2+(y_init-MIOPos(2))^2);
    %dist2crash = 40;
    %T_f = abs(dist2crash/(MIOVel-V_i));
    T_f = 3;
    P = [1, T_i, T_i^2, T_i^3, T_i^4, T_i^5;
         0, 1, 2*T_i, 3*T_i^2, 4*T_i^3, 5*T_i^4;
         0, 0, 2, 6*T_i, 12*T_i^2, 20*T_i^3;
         1, T_f, T_f^2, T_f^3, T_f^4, T_f^5;
         0, 1, 2*T_f, 3*T_f^2, 4*T_f^3, 5*T_f^4;
         0, 0, 2, 6*T_f, 12*T_f^2, 20*T_f^3];

%     mtang4 = (yq(1,index+2)-yq(1,index+1))/(xq(1,index+2)-xq(1,index+1));

    Vx_i = vd_n*cos(theta4); 
    Vy_i = vd_n*sin(theta4); 
    Ax_i = ad_n*cos(theta4)-vd_n*sin(theta4)*wd_n; 
    Ay_i = ad_n*sin(theta4)+vd_n*cos(theta4)*wd_n;

%     if(xq(index+2)-xq(index+1)<0)
%         theta_4 = pi + atan(mtang4);
%     else
%         theta_4 = atan(mtang4);
%     end

    theta_4 =0;
    Vx_f = V_f*cos(theta_4); % curvature angle
    Vy_f = V_f*sin(theta_4);
    Ax_f = A_f*cos(theta_4)-V_f*sin(theta_4)*W_f;
    Ay_f = A_f*sin(theta_4)+V_f*cos(theta_4)*W_f;

    g1 = [x_init; Vx_i; Ax_i; xf; Vx_f; Ax_f];
    g2 = [y_init; Vy_i; Ay_i; yf; Vy_f; Ay_f];

    a_coeff = P\g1;
    b_coeff = P\g2;
    
    td = T_i;
    scatter(x_init,y_init,'go')
    hold on; 
    scatter(xf,yf,'ro')
    hold on;
    
    for f = 1:(num_foc_t+1)
        xd(f,1) = [1,td,td^2,td^3,td^4,td^5]*a_coeff 
        yd(f,1) = [1,td,td^2,td^3,td^4,td^5]*b_coeff
        td = td + (T_f - T_i)/num_foc_t;
        scatter(xd(f,1),yd(f,1),'y.');
    end

LCinProgress = 1;

% hold on;
end

== stateflow chart vehicle_hostmodel_2022b_v11/Behavioural Planner/Collision Avoidance ==
  state Stop
    en:
    Brake = 1;
  state Start
    en:
    Stuck = 0;
    ACC = 0;
    LaneChangeCmd = 0;
    %VelCmd = CurrentVelCmd;
  state Follow
    en:
    ACC = 1;
    Brake = 0;
  state LaneChange
    en:
    LaneChangeCmd = 1;
    ACC=0;
  Stop -> Follow : [EgoSpeed<0.1]
  Follow -> Stop [order 4] : [D2O < 20 && EgoSpeed > 2]
  (default) -> Start
  Follow -> LaneChange [order 2] : [LC_ACC==1]
  Start -> Follow : [ObjAhead == 1]
  Follow -> Start [order 3] : [ObjAhead == 0]
  LaneChange -> Start : [LaneChanged == 1]
  Follow -> Follow [order 1] : [(EgoSpeed <= MinSpeed) && after(WaitTime,sec)]{Stuck = 1;}
  data: Stuck local; ACC output; WaitTime input; ObjAhead input; MinSpeed input; LaneAvailable input; EgoSpeed input; LaneChanged input; LC_ACC input; LaneChangeCmd output; Brake output; D2O input

== matlab function vehicle_hostmodel_2022b_v11/Behavioural Planner/Destination ==
  data: u input; y output
function y = fcn(u)

y = [u(99,1) u(99,2)];
end

== matlab function vehicle_hostmodel_2022b_v11/Controllers/MATLAB Function2 ==
  data: v input; RefVelCmd output; curvature input
function RefVelCmd = fcn(v,curvature)

    if abs(curvature) >= 0 && abs(curvature) <= 1e-2
        RefVelCmd = v;
    else
        r = 1/abs(curvature);
        RefVelCmd = min(v,sqrt(9.81*r*.2));
    end

== matlab function vehicle_hostmodel_2022b_v11/Vehicle Dynamics/Info2ActorState/MATLAB Function1 ==
  data: Xdot input; Velocity output; Ydot input; Zdot input
function Velocity = fcn(Xdot, Ydot, Zdot)

Velocity = [Xdot Ydot, Zdot];

== stateflow chart vehicle_hostmodel_2022b_v11/Behavioural Planner/Emergency Stop ==
  state EmergencyCheck
    en:
    EStop = 0;
  state Pullover
    en:
    EStop=1;
  state Stop
    en:
    EStop=2;
  Pullover -> EmergencyCheck : [TechFailure == 0]
  (default) -> EmergencyCheck
  EmergencyCheck -> Pullover [order 1] : [TechFailure == 1]
  EmergencyCheck -> Stop [order 2] : [D2O<=1]
  Stop -> EmergencyCheck : [D2O > 2]
  data: D2O input; TechFailure input; EStop output

== matlab function vehicle_hostmodel_2022b_v11/MATLAB Function ==
  data: ttc output; dist output; left output; right output; LL_avail output; RL_avail output; tend2stay output; ego input; act input; LaneBounds input; RoadSpeed input; ego_vel output; stay output; LL_Change output; RL_Change output; y_lane output; LCinProgress input
function [ttc,dist,left,right,LL_avail,RL_avail,tend2stay,ego_vel,stay,LL_Change,RL_Change,y_lane] = fcn(ego,act,LaneBounds,RoadSpeed, LCinProgress)                       


%% Major tasks to look into

% Check the performance while transitioning into another lane 
% Lane change output when the ego on extreme lanes.
% Develop code to handle lane changes on road curvatures
% Integrate with the trajectory generation and check the perfomance
% Convert the code to ego vehicle coordinates


%%
%define some parameters
r_c = 20; %range considered to MIOs
t_min =  2;

num_actors = length(act.Actors);
%num_lanes = length(LaneBounds.LaneBoundaries)-1;


%% Using sensor data 
% TracksNum = Tracking.NumTracks;
% 
% 
% for t = 1:TracksNum
%     ObjectID(t) = Tracking.Tracks(t).ObjectClassID;
%     TrackPos(:,t) = Tracking.Tracks(t).State(1:2:5);
%     TrackVel(:,t) = Tracking.Tracks(t).State(2:2:6);

%% ego position and  velocity magnitude
ego_pos = ego.Position;
ego_vel = ego.Velocity(1);  % velocity

%ttc: (array) : agent.relative position / abs(relative velocity)
ttc = zeros(1,num_actors);
left = zeros(1,num_actors);
right = zeros(1,num_actors);

dist =  zeros(1,num_actors);
tend2stay=1;

%%
y_lane = zeros(1,length(LaneBounds.LaneBoundaries))

for l=1:length(y_lane)
    y_lane(l)=LaneBounds.LaneBoundaries(l).Coordinates(end,2)
end

%%
for i= 1:num_actors

    % Grab actor positions and velocities
    actor_pos = act.Actors(i).Position;   
    actor_vel = act.Actors(i).Velocity(1);  % x-component velocity

    %relative velocity of the agent
    rel_vel = actor_vel - ego_vel;


    %% Check if the actor is within a r_c range. If it is out of range, pass lane change as '1' automatically.

   dist(i) = norm([actor_pos(1) actor_pos(2)]-[ego_pos(1) ego_pos(2)]);
        
    if dist(i) > r_c
        left(i)=1;
        right(i)=1;
        continue
    end

    %% Check if the actor is in the same lane as that of ego

    % If the actor and ego are in the same lane, it is considered a lead/following vehicle in the same lane and by defualt, the lane change flag is 1.

    if (actor_pos(2)< (ego_pos(2)+0.5) && actor_pos(2) > (ego_pos(2)-0.5))
        if (rel_vel < 0 && ego_vel < (RoadSpeed+5) && actor_pos(1) > ego_pos(1) )
            left(i) =1;
            right(i)=1;
            tend2stay=0;        % we need to incorporate too slow condition even when the relative velocity is greater than 0.

        elseif (rel_vel < 0 && ego_vel < (RoadSpeed+5) && actor_pos(1) < ego_pos(1) )
            left(i) =1;
            right(i)=1;
            tend2stay=1;
        end

        continue
    end

    
    %% calculate ttc for the rest of the vehicles


    ttc(i) = (actor_pos(1)-ego_pos(1))/abs(rel_vel);

    % checking conditions for other surrounding actors

    % all actors on the left lane of the ego vehicle
%%
    if actor_pos(2)-ego_pos(2) > 0  

        if and(rel_vel>0, ttc(i) > t_min)  % target vehicles on the front of ego vehicle (any lane)
    
            left(i)=1; 
            right(i)=1;
    
        elseif (ttc(i)<0 && rel_vel<0 && abs(ttc(i)) > t_min)    % target vehicle on the back of ego vehicle (ttc<0) (any lane)
            left(i) =1;
            right(i)=1;
    
        else 
            left(i) =0;
            right(i)=1;
    
        end

    % all actors on the right lane of the ego vehicle

    elseif actor_pos(2)-ego_pos(2) < 0
         
        if and(rel_vel>0, ttc(i) > t_min)  % target vehicles on the front of ego vehicle (any lane)
    
            left(i)=1;
            right(i)=1;
    
        elseif (ttc(i)<0 && rel_vel<0 && abs(ttc(i)) > t_min)    % target vehicle on the back of ego vehicle (ttc<0) (any lane)
            left(i) =1;
            right(i)=1;
    
        else 
            left(i) =1;
            right(i)=0;
    
        end
    end
%%

end

%% check if the vehicle is in the extreme end lanes

    if ego_pos(2)<y_lane(1) && ego_pos(2)>y_lane(2)

        LL=0; RL=1;
    elseif ego_pos(2) > y_lane(end) && ego_pos(2) < y_lane(end-1)
        RL=0; LL=1;
    else 

        RL=1;LL=1;
    end

%%
LL_avail = all(left) %&& LL;

RL_avail = all(right) %&& RL               %&& ~lcLeft ; this can be decided later 


%% final commands

stay = tend2stay || ~(tend2stay || LL_avail || RL_avail);
LL_Change =  ~tend2stay && LL_avail ;

RL_Change =  ~tend2stay && RL_avail && ~LL_Change ;
LCFlag = ~stay;
if LCFlag && LCinProgress
    LCFlag = false;
    stay = ~LCFlag;
end

%% 






end

== matlab function vehicle_hostmodel_2022b_v11/Vehicle Dynamics/Info2ActorState/MATLAB Function2 ==
  data: aX input; Acceleration output; aY input; aZ input
function Acceleration = fcn(aX, aY, aZ)

Acceleration = [aX aY, aZ];

== matlab function vehicle_hostmodel_2022b_v11/Vehicle Dynamics/Info2ActorState/MATLAB Function3 ==
  data: phiDot input; AngularVelocity output; thetaDot input; psiDot input
function AngularVelocity = fcn(phiDot, thetaDot, psiDot)

AngularVelocity = [phiDot thetaDot, psiDot];
